simulink model "DBX_aero_parametric"  (R2015b)
settings: Solver=VariableStepAuto  StartTime=0.0  StopTime=10.0  RelTol=1e-3
undefined symbols (not defined in the file or in its folder): DBX_aero_param
libraries: simulink x28
settings Model: Creator=DTorres  LastModifiedBy=DTorres

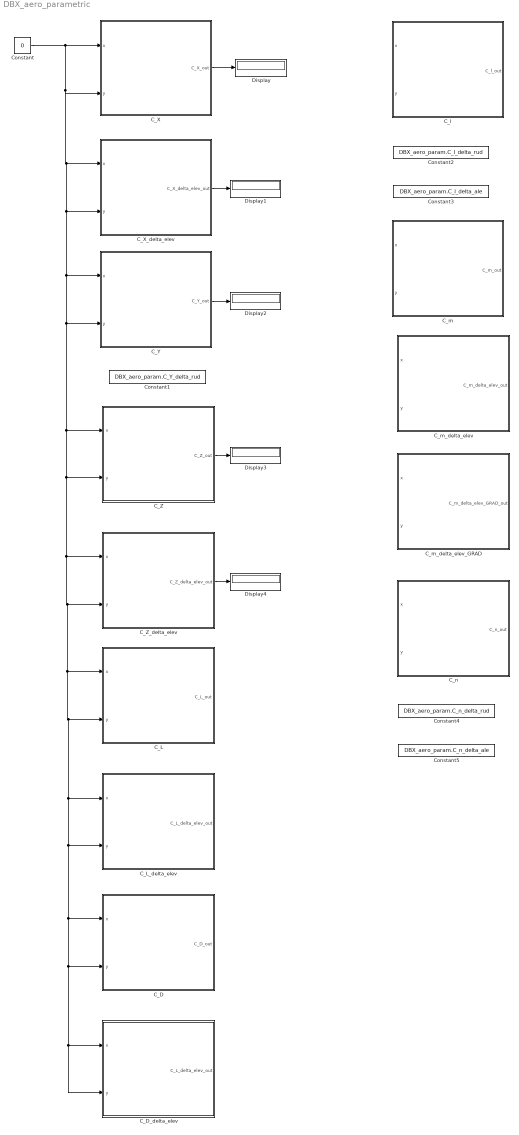
== system DBX_aero_parametric ==
  C_D : Subsystem
  C_D_delta_elev : Subsystem
  C_L : Subsystem
  C_L_delta_elev : Subsystem
  C_X : Subsystem
  C_X_delta_elev : Subsystem
  C_Y : Subsystem
  C_Z : Subsystem
  C_Z_delta_elev : Subsystem
  C_l : Subsystem
  C_m : Subsystem
  C_m_delta_elev : Subsystem
  C_m_delta_elev_GRAD : Subsystem
  C_n : Subsystem
  Constant : Constant  Value=0
  Constant1 : Constant  Value=DBX_aero_param.C_Y_delta_rud
  Constant2 : Constant  Value=DBX_aero_param.C_l_delta_rud
  Constant3 : Constant  Value=DBX_aero_param.C_l_delta_ale
  Constant4 : Constant  Value=DBX_aero_param.C_n_delta_rud
  Constant5 : Constant  Value=DBX_aero_param.C_n_delta_ale
  Display{,1..4} (5 alike) : Display
  wires:
  Constant/1 -> C_D_delta_elev/2(y), C_D_delta_elev/1(x), C_D/2(y), C_D/1(x), C_L_delta_elev/2(y), C_L_delta_elev/1(x), C_L/2(y), C_L/1(x), C_Z_delta_elev/2(y), C_Z_delta_elev/1(x), C_Z/2(y), C_Z/1(x), C_Y/2(y), C_Y/1(x), C_X_delta_elev/2(y), C_X_delta_elev/1(x), C_X/2(y), C_X/1(x)
  C_X/1(C_X_out) -> Display/1
  C_X_delta_elev/1(C_X_delta_elev_out) -> Display1/1
  C_Y/1(C_Y_out) -> Display2/1
  C_Z/1(C_Z_out) -> Display3/1
  C_Z_delta_elev/1(C_Z_delta_elev_out) -> Display4/1

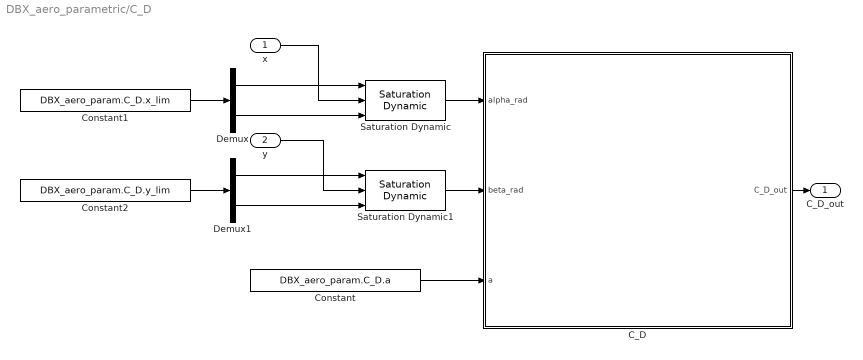
== system DBX_aero_parametric/C_D ==
  x : Inport
  y : Inport  Port=2
  C_D : MATLAB Function
  Constant : Constant  Value=DBX_aero_param.C_D.a
  Constant1 : Constant  Value=DBX_aero_param.C_D.x_lim
  Constant2 : Constant  Value=DBX_aero_param.C_D.y_lim
  Demux : Demux  Outputs=2
  Demux1 : Demux  Outputs=2
  Saturation Dynamic : simulink/Discontinuities/Saturation Dynamic  OutMin=[]  OutMax=[]  OutDataTypeStr=Inherit: Same as second input  OutDataType=fixdt(1, 16)  OutScaling=2^-10  DoSatur=off
  Saturation Dynamic1 : simulink/Discontinuities/Saturation Dynamic  OutMin=[]  OutMax=[]  OutDataTypeStr=Inherit: Same as second input  OutDataType=fixdt(1, 16)  OutScaling=2^-10  DoSatur=off
  C_D_out : Outport
  wires:
  Demux/1 -> Saturation Dynamic/1
  y/1 -> Saturation Dynamic1/2
  Demux/2 -> Saturation Dynamic/3
  Constant1/1 -> Demux/1
  x/1 -> Saturation Dynamic/2
  Demux1/2 -> Saturation Dynamic1/3
  Saturation Dynamic/1 -> C_D/1(alpha_rad)
  Demux1/1 -> Saturation Dynamic1/1
  Saturation Dynamic1/1 -> C_D/2(beta_rad)
  Constant2/1 -> Demux1/1
  C_D/1(C_D_out) -> C_D_out/1
  Constant/1 -> C_D/3(a)

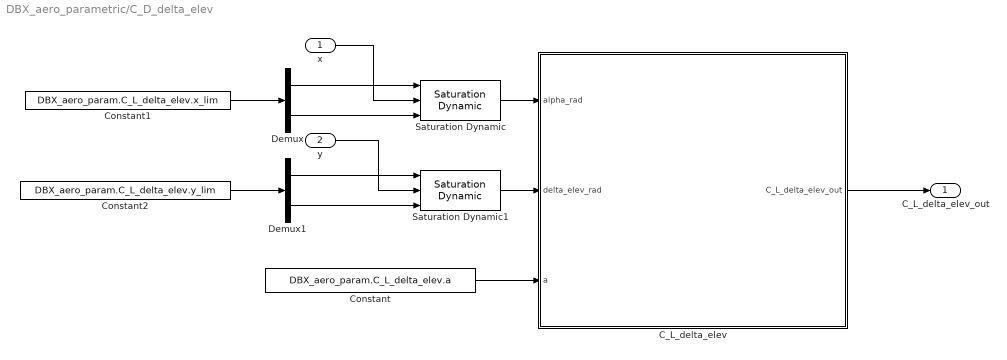
== system DBX_aero_parametric/C_D_delta_elev ==
  x : Inport
  y : Inport  Port=2
  C_L_delta_elev : MATLAB Function
  Constant : Constant  Value=DBX_aero_param.C_L_delta_elev.a
  Constant1 : Constant  Value=DBX_aero_param.C_L_delta_elev.x_lim
  Constant2 : Constant  Value=DBX_aero_param.C_L_delta_elev.y_lim
  Demux : Demux  Outputs=2
  Demux1 : Demux  Outputs=2
  Saturation Dynamic : simulink/Discontinuities/Saturation Dynamic  OutMin=[]  OutMax=[]  OutDataTypeStr=Inherit: Same as second input  OutDataType=fixdt(1, 16)  OutScaling=2^-10  DoSatur=off
  Saturation Dynamic1 : simulink/Discontinuities/Saturation Dynamic  OutMin=[]  OutMax=[]  OutDataTypeStr=Inherit: Same as second input  OutDataType=fixdt(1, 16)  OutScaling=2^-10  DoSatur=off
  C_L_delta_elev_out : Outport
  wires:
  Constant/1 -> C_L_delta_elev/3(a)
  C_L_delta_elev/1(C_L_delta_elev_out) -> C_L_delta_elev_out/1
  Constant2/1 -> Demux1/1
  Saturation Dynamic1/1 -> C_L_delta_elev/2(delta_elev_rad)
  Demux1/1 -> Saturation Dynamic1/1
  Saturation Dynamic/1 -> C_L_delta_elev/1(alpha_rad)
  Demux1/2 -> Saturation Dynamic1/3
  x/1 -> Saturation Dynamic/2
  Constant1/1 -> Demux/1
  Demux/2 -> Saturation Dynamic/3
  y/1 -> Saturation Dynamic1/2
  Demux/1 -> Saturation Dynamic/1

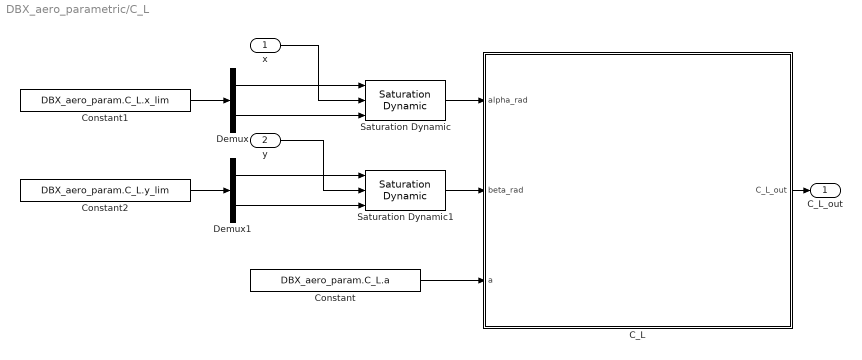
== system DBX_aero_parametric/C_L ==
  x : Inport
  y : Inport  Port=2
  C_L : MATLAB Function
  Constant : Constant  Value=DBX_aero_param.C_L.a
  Constant1 : Constant  Value=DBX_aero_param.C_L.x_lim
  Constant2 : Constant  Value=DBX_aero_param.C_L.y_lim
  Demux : Demux  Outputs=2
  Demux1 : Demux  Outputs=2
  Saturation Dynamic : simulink/Discontinuities/Saturation Dynamic  OutMin=[]  OutMax=[]  OutDataTypeStr=Inherit: Same as second input  OutDataType=fixdt(1, 16)  OutScaling=2^-10  DoSatur=off
  Saturation Dynamic1 : simulink/Discontinuities/Saturation Dynamic  OutMin=[]  OutMax=[]  OutDataTypeStr=Inherit: Same as second input  OutDataType=fixdt(1, 16)  OutScaling=2^-10  DoSatur=off
  C_L_out : Outport
  wires:
  Constant/1 -> C_L/3(a)
  C_L/1(C_L_out) -> C_L_out/1
  Constant2/1 -> Demux1/1
  Saturation Dynamic1/1 -> C_L/2(beta_rad)
  Demux1/1 -> Saturation Dynamic1/1
  Saturation Dynamic/1 -> C_L/1(alpha_rad)
  Demux1/2 -> Saturation Dynamic1/3
  x/1 -> Saturation Dynamic/2
  Constant1/1 -> Demux/1
  Demux/2 -> Saturation Dynamic/3
  y/1 -> Saturation Dynamic1/2
  Demux/1 -> Saturation Dynamic/1

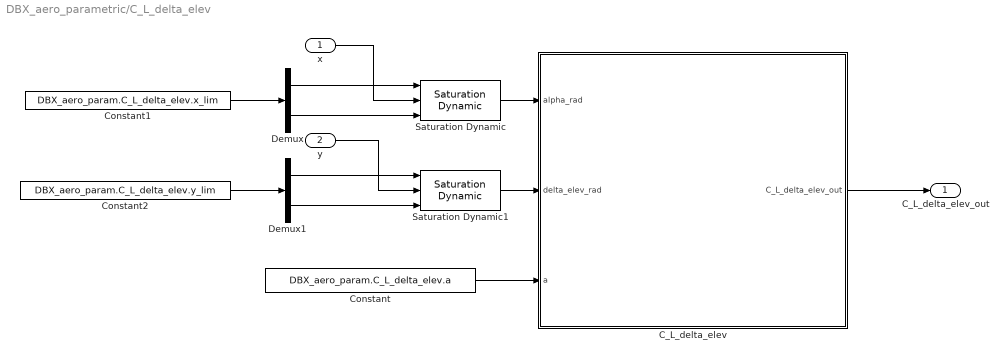
== system DBX_aero_parametric/C_L_delta_elev ==
  x : Inport
  y : Inport  Port=2
  C_L_delta_elev : MATLAB Function
  Constant : Constant  Value=DBX_aero_param.C_L_delta_elev.a
  Constant1 : Constant  Value=DBX_aero_param.C_L_delta_elev.x_lim
  Constant2 : Constant  Value=DBX_aero_param.C_L_delta_elev.y_lim
  Demux : Demux  Outputs=2
  Demux1 : Demux  Outputs=2
  Saturation Dynamic : simulink/Discontinuities/Saturation Dynamic  OutMin=[]  OutMax=[]  OutDataTypeStr=Inherit: Same as second input  OutDataType=fixdt(1, 16)  OutScaling=2^-10  DoSatur=off
  Saturation Dynamic1 : simulink/Discontinuities/Saturation Dynamic  OutMin=[]  OutMax=[]  OutDataTypeStr=Inherit: Same as second input  OutDataType=fixdt(1, 16)  OutScaling=2^-10  DoSatur=off
  C_L_delta_elev_out : Outport
  wires:
  Demux/1 -> Saturation Dynamic/1
  y/1 -> Saturation Dynamic1/2
  Demux/2 -> Saturation Dynamic/3
  Constant1/1 -> Demux/1
  x/1 -> Saturation Dynamic/2
  Demux1/2 -> Saturation Dynamic1/3
  Saturation Dynamic/1 -> C_L_delta_elev/1(alpha_rad)
  Demux1/1 -> Saturation Dynamic1/1
  Saturation Dynamic1/1 -> C_L_delta_elev/2(delta_elev_rad)
  Constant2/1 -> Demux1/1
  C_L_delta_elev/1(C_L_delta_elev_out) -> C_L_delta_elev_out/1
  Constant/1 -> C_L_delta_elev/3(a)

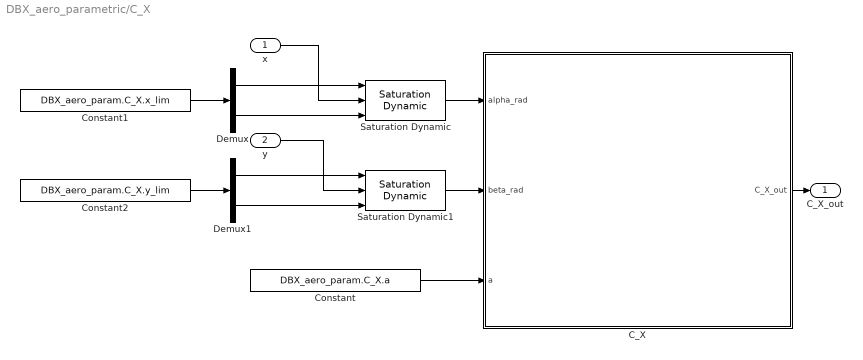
== system DBX_aero_parametric/C_X ==
  x : Inport
  y : Inport  Port=2
  C_X : MATLAB Function
  Constant : Constant  Value=DBX_aero_param.C_X.a
  Constant1 : Constant  Value=DBX_aero_param.C_X.x_lim
  Constant2 : Constant  Value=DBX_aero_param.C_X.y_lim
  Demux : Demux  Outputs=2
  Demux1 : Demux  Outputs=2
  Saturation Dynamic : simulink/Discontinuities/Saturation Dynamic  OutMin=[]  OutMax=[]  OutDataTypeStr=Inherit: Same as second input  OutDataType=fixdt(1, 16)  OutScaling=2^-10  DoSatur=off
  Saturation Dynamic1 : simulink/Discontinuities/Saturation Dynamic  OutMin=[]  OutMax=[]  OutDataTypeStr=Inherit: Same as second input  OutDataType=fixdt(1, 16)  OutScaling=2^-10  DoSatur=off
  C_X_out : Outport
  wires:
  Constant/1 -> C_X/3(a)
  C_X/1(C_X_out) -> C_X_out/1
  Constant2/1 -> Demux1/1
  Saturation Dynamic1/1 -> C_X/2(beta_rad)
  Demux1/1 -> Saturation Dynamic1/1
  Saturation Dynamic/1 -> C_X/1(alpha_rad)
  Demux1/2 -> Saturation Dynamic1/3
  x/1 -> Saturation Dynamic/2
  Constant1/1 -> Demux/1
  Demux/2 -> Saturation Dynamic/3
  y/1 -> Saturation Dynamic1/2
  Demux/1 -> Saturation Dynamic/1

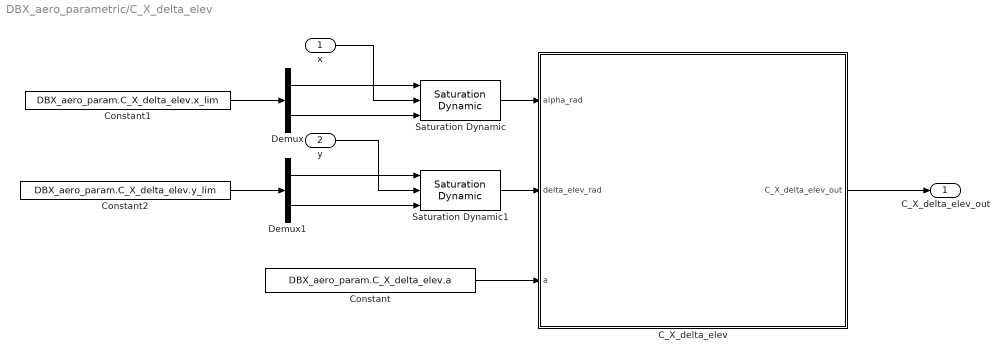
== system DBX_aero_parametric/C_X_delta_elev ==
  x : Inport
  y : Inport  Port=2
  C_X_delta_elev : MATLAB Function
  Constant : Constant  Value=DBX_aero_param.C_X_delta_elev.a
  Constant1 : Constant  Value=DBX_aero_param.C_X_delta_elev.x_lim
  Constant2 : Constant  Value=DBX_aero_param.C_X_delta_elev.y_lim
  Demux : Demux  Outputs=2
  Demux1 : Demux  Outputs=2
  Saturation Dynamic : simulink/Discontinuities/Saturation Dynamic  OutMin=[]  OutMax=[]  OutDataTypeStr=Inherit: Same as second input  OutDataType=fixdt(1, 16)  OutScaling=2^-10  DoSatur=off
  Saturation Dynamic1 : simulink/Discontinuities/Saturation Dynamic  OutMin=[]  OutMax=[]  OutDataTypeStr=Inherit: Same as second input  OutDataType=fixdt(1, 16)  OutScaling=2^-10  DoSatur=off
  C_X_delta_elev_out : Outport
  wires:
  Demux/1 -> Saturation Dynamic/1
  y/1 -> Saturation Dynamic1/2
  Demux/2 -> Saturation Dynamic/3
  Constant1/1 -> Demux/1
  x/1 -> Saturation Dynamic/2
  Demux1/2 -> Saturation Dynamic1/3
  Saturation Dynamic/1 -> C_X_delta_elev/1(alpha_rad)
  Demux1/1 -> Saturation Dynamic1/1
  Saturation Dynamic1/1 -> C_X_delta_elev/2(delta_elev_rad)
  Constant2/1 -> Demux1/1
  C_X_delta_elev/1(C_X_delta_elev_out) -> C_X_delta_elev_out/1
  Constant/1 -> C_X_delta_elev/3(a)

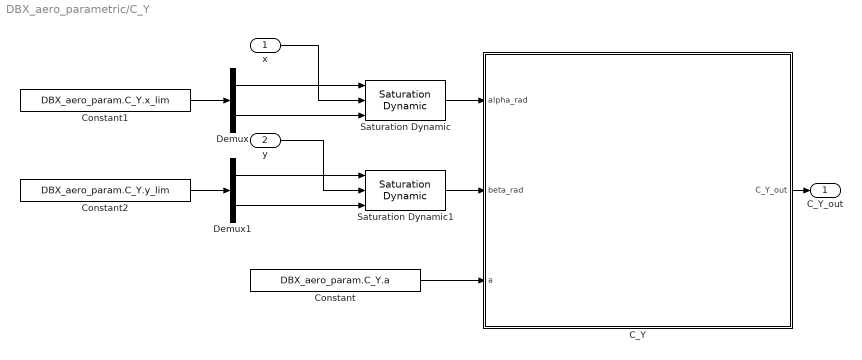
== system DBX_aero_parametric/C_Y ==
  x : Inport
  y : Inport  Port=2
  C_Y : MATLAB Function
  Constant : Constant  Value=DBX_aero_param.C_Y.a
  Constant1 : Constant  Value=DBX_aero_param.C_Y.x_lim
  Constant2 : Constant  Value=DBX_aero_param.C_Y.y_lim
  Demux : Demux  Outputs=2
  Demux1 : Demux  Outputs=2
  Saturation Dynamic : simulink/Discontinuities/Saturation Dynamic  OutMin=[]  OutMax=[]  OutDataTypeStr=Inherit: Same as second input  OutDataType=fixdt(1, 16)  OutScaling=2^-10  DoSatur=off
  Saturation Dynamic1 : simulink/Discontinuities/Saturation Dynamic  OutMin=[]  OutMax=[]  OutDataTypeStr=Inherit: Same as second input  OutDataType=fixdt(1, 16)  OutScaling=2^-10  DoSatur=off
  C_Y_out : Outport
  wires:
  Demux/1 -> Saturation Dynamic/1
  y/1 -> Saturation Dynamic1/2
  Demux/2 -> Saturation Dynamic/3
  Constant1/1 -> Demux/1
  x/1 -> Saturation Dynamic/2
  Demux1/2 -> Saturation Dynamic1/3
  Saturation Dynamic/1 -> C_Y/1(alpha_rad)
  Demux1/1 -> Saturation Dynamic1/1
  Saturation Dynamic1/1 -> C_Y/2(beta_rad)
  Constant2/1 -> Demux1/1
  C_Y/1(C_Y_out) -> C_Y_out/1
  Constant/1 -> C_Y/3(a)

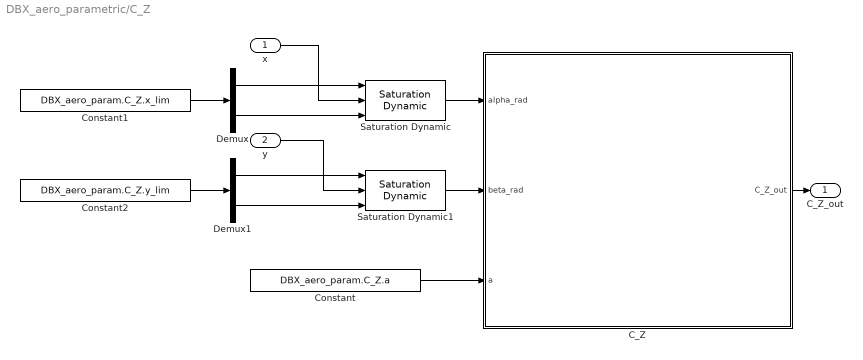
== system DBX_aero_parametric/C_Z ==
  x : Inport
  y : Inport  Port=2
  C_Z : MATLAB Function
  Constant : Constant  Value=DBX_aero_param.C_Z.a
  Constant1 : Constant  Value=DBX_aero_param.C_Z.x_lim
  Constant2 : Constant  Value=DBX_aero_param.C_Z.y_lim
  Demux : Demux  Outputs=2
  Demux1 : Demux  Outputs=2
  Saturation Dynamic : simulink/Discontinuities/Saturation Dynamic  OutMin=[]  OutMax=[]  OutDataTypeStr=Inherit: Same as second input  OutDataType=fixdt(1, 16)  OutScaling=2^-10  DoSatur=off
  Saturation Dynamic1 : simulink/Discontinuities/Saturation Dynamic  OutMin=[]  OutMax=[]  OutDataTypeStr=Inherit: Same as second input  OutDataType=fixdt(1, 16)  OutScaling=2^-10  DoSatur=off
  C_Z_out : Outport
  wires:
  Demux/1 -> Saturation Dynamic/1
  y/1 -> Saturation Dynamic1/2
  Demux/2 -> Saturation Dynamic/3
  Constant1/1 -> Demux/1
  x/1 -> Saturation Dynamic/2
  Demux1/2 -> Saturation Dynamic1/3
  Saturation Dynamic/1 -> C_Z/1(alpha_rad)
  Demux1/1 -> Saturation Dynamic1/1
  Saturation Dynamic1/1 -> C_Z/2(beta_rad)
  Constant2/1 -> Demux1/1
  C_Z/1(C_Z_out) -> C_Z_out/1
  Constant/1 -> C_Z/3(a)

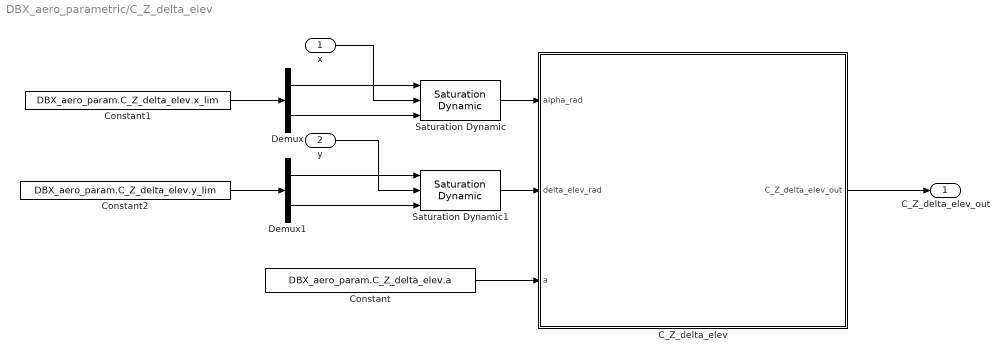
== system DBX_aero_parametric/C_Z_delta_elev ==
  x : Inport
  y : Inport  Port=2
  C_Z_delta_elev : MATLAB Function
  Constant : Constant  Value=DBX_aero_param.C_Z_delta_elev.a
  Constant1 : Constant  Value=DBX_aero_param.C_Z_delta_elev.x_lim
  Constant2 : Constant  Value=DBX_aero_param.C_Z_delta_elev.y_lim
  Demux : Demux  Outputs=2
  Demux1 : Demux  Outputs=2
  Saturation Dynamic : simulink/Discontinuities/Saturation Dynamic  OutMin=[]  OutMax=[]  OutDataTypeStr=Inherit: Same as second input  OutDataType=fixdt(1, 16)  OutScaling=2^-10  DoSatur=off
  Saturation Dynamic1 : simulink/Discontinuities/Saturation Dynamic  OutMin=[]  OutMax=[]  OutDataTypeStr=Inherit: Same as second input  OutDataType=fixdt(1, 16)  OutScaling=2^-10  DoSatur=off
  C_Z_delta_elev_out : Outport
  wires:
  Constant/1 -> C_Z_delta_elev/3(a)
  C_Z_delta_elev/1(C_Z_delta_elev_out) -> C_Z_delta_elev_out/1
  Constant2/1 -> Demux1/1
  Saturation Dynamic1/1 -> C_Z_delta_elev/2(delta_elev_rad)
  Demux1/1 -> Saturation Dynamic1/1
  Saturation Dynamic/1 -> C_Z_delta_elev/1(alpha_rad)
  Demux1/2 -> Saturation Dynamic1/3
  x/1 -> Saturation Dynamic/2
  Constant1/1 -> Demux/1
  Demux/2 -> Saturation Dynamic/3
  y/1 -> Saturation Dynamic1/2
  Demux/1 -> Saturation Dynamic/1

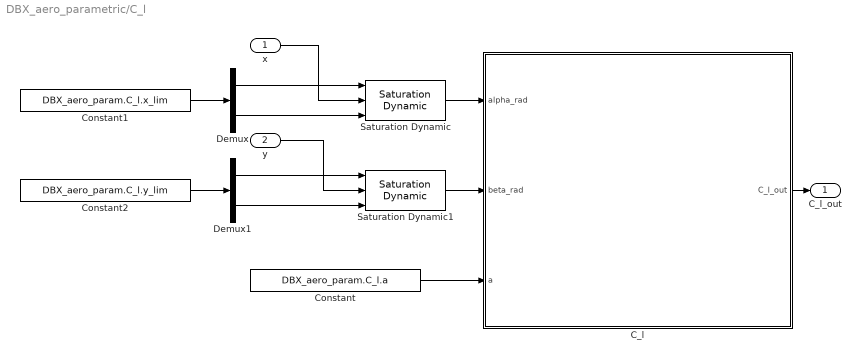
== system DBX_aero_parametric/C_l ==
  x : Inport
  y : Inport  Port=2
  C_l : MATLAB Function
  Constant : Constant  Value=DBX_aero_param.C_l.a
  Constant1 : Constant  Value=DBX_aero_param.C_l.x_lim
  Constant2 : Constant  Value=DBX_aero_param.C_l.y_lim
  Demux : Demux  Outputs=2
  Demux1 : Demux  Outputs=2
  Saturation Dynamic : simulink/Discontinuities/Saturation Dynamic  OutMin=[]  OutMax=[]  OutDataTypeStr=Inherit: Same as second input  OutDataType=fixdt(1, 16)  OutScaling=2^-10  DoSatur=off
  Saturation Dynamic1 : simulink/Discontinuities/Saturation Dynamic  OutMin=[]  OutMax=[]  OutDataTypeStr=Inherit: Same as second input  OutDataType=fixdt(1, 16)  OutScaling=2^-10  DoSatur=off
  C_l_out : Outport
  wires:
  Demux/1 -> Saturation Dynamic/1
  y/1 -> Saturation Dynamic1/2
  Demux/2 -> Saturation Dynamic/3
  Constant1/1 -> Demux/1
  x/1 -> Saturation Dynamic/2
  Demux1/2 -> Saturation Dynamic1/3
  Saturation Dynamic/1 -> C_l/1(alpha_rad)
  Demux1/1 -> Saturation Dynamic1/1
  Saturation Dynamic1/1 -> C_l/2(beta_rad)
  Constant2/1 -> Demux1/1
  C_l/1(C_l_out) -> C_l_out/1
  Constant/1 -> C_l/3(a)

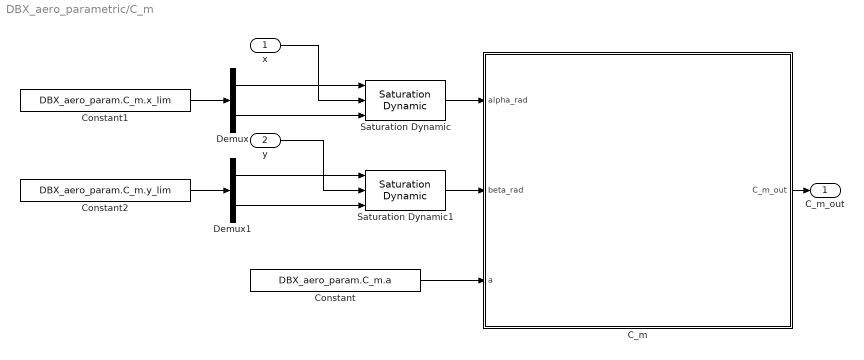
== system DBX_aero_parametric/C_m ==
  x : Inport
  y : Inport  Port=2
  C_m : MATLAB Function
  Constant : Constant  Value=DBX_aero_param.C_m.a
  Constant1 : Constant  Value=DBX_aero_param.C_m.x_lim
  Constant2 : Constant  Value=DBX_aero_param.C_m.y_lim
  Demux : Demux  Outputs=2
  Demux1 : Demux  Outputs=2
  Saturation Dynamic : simulink/Discontinuities/Saturation Dynamic  OutMin=[]  OutMax=[]  OutDataTypeStr=Inherit: Same as second input  OutDataType=fixdt(1, 16)  OutScaling=2^-10  DoSatur=off
  Saturation Dynamic1 : simulink/Discontinuities/Saturation Dynamic  OutMin=[]  OutMax=[]  OutDataTypeStr=Inherit: Same as second input  OutDataType=fixdt(1, 16)  OutScaling=2^-10  DoSatur=off
  C_m_out : Outport
  wires:
  Demux/1 -> Saturation Dynamic/1
  y/1 -> Saturation Dynamic1/2
  Demux/2 -> Saturation Dynamic/3
  Constant1/1 -> Demux/1
  x/1 -> Saturation Dynamic/2
  Demux1/2 -> Saturation Dynamic1/3
  Saturation Dynamic/1 -> C_m/1(alpha_rad)
  Demux1/1 -> Saturation Dynamic1/1
  Saturation Dynamic1/1 -> C_m/2(beta_rad)
  Constant2/1 -> Demux1/1
  C_m/1(C_m_out) -> C_m_out/1
  Constant/1 -> C_m/3(a)

== system DBX_aero_parametric/C_m_delta_elev ==
  x : Inport
  y : Inport  Port=2
  C_m_delta_elev : MATLAB Function
  Constant : Constant  Value=DBX_aero_param.C_m_delta_elev.a
  Constant1 : Constant  Value=DBX_aero_param.C_m_delta_elev.x_lim
  Constant2 : Constant  Value=DBX_aero_param.C_m_delta_elev.y_lim
  Demux : Demux  Outputs=2
  Demux1 : Demux  Outputs=2
  Saturation Dynamic : simulink/Discontinuities/Saturation Dynamic  OutMin=[]  OutMax=[]  OutDataTypeStr=Inherit: Same as second input  OutDataType=fixdt(1, 16)  OutScaling=2^-10  DoSatur=off
  Saturation Dynamic1 : simulink/Discontinuities/Saturation Dynamic  OutMin=[]  OutMax=[]  OutDataTypeStr=Inherit: Same as second input  OutDataType=fixdt(1, 16)  OutScaling=2^-10  DoSatur=off
  C_m_delta_elev_out : Outport
  wires:
  Constant/1 -> C_m_delta_elev/3(a)
  C_m_delta_elev/1(C_m_delta_elev_out) -> C_m_delta_elev_out/1
  Constant2/1 -> Demux1/1
  Saturation Dynamic1/1 -> C_m_delta_elev/2(delta_elev_rad)
  Demux1/1 -> Saturation Dynamic1/1
  Saturation Dynamic/1 -> C_m_delta_elev/1(alpha_rad)
  Demux1/2 -> Saturation Dynamic1/3
  x/1 -> Saturation Dynamic/2
  Constant1/1 -> Demux/1
  Demux/2 -> Saturation Dynamic/3
  y/1 -> Saturation Dynamic1/2
  Demux/1 -> Saturation Dynamic/1

== system DBX_aero_parametric/C_m_delta_elev_GRAD ==
  x : Inport
  y : Inport  Port=2
  C_m_delta_elev_GRAD : MATLAB Function
  Constant : Constant  Value=DBX_aero_param.C_m_delta_elev_GRAD.a
  Constant1 : Constant  Value=DBX_aero_param.C_m_delta_elev_GRAD.x_lim
  Constant2 : Constant  Value=DBX_aero_param.C_m_delta_elev_GRAD.y_lim
  Demux : Demux  Outputs=2
  Demux1 : Demux  Outputs=2
  Saturation Dynamic : simulink/Discontinuities/Saturation Dynamic  OutMin=[]  OutMax=[]  OutDataTypeStr=Inherit: Same as second input  OutDataType=fixdt(1, 16)  OutScaling=2^-10  DoSatur=off
  Saturation Dynamic1 : simulink/Discontinuities/Saturation Dynamic  OutMin=[]  OutMax=[]  OutDataTypeStr=Inherit: Same as second input  OutDataType=fixdt(1, 16)  OutScaling=2^-10  DoSatur=off
  C_m_delta_elev_GRAD_out : Outport
  wires:
  Demux/1 -> Saturation Dynamic/1
  y/1 -> Saturation Dynamic1/2
  Demux/2 -> Saturation Dynamic/3
  Constant1/1 -> Demux/1
  x/1 -> Saturation Dynamic/2
  Demux1/2 -> Saturation Dynamic1/3
  Saturation Dynamic/1 -> C_m_delta_elev_GRAD/1(alpha_rad)
  Demux1/1 -> Saturation Dynamic1/1
  Saturation Dynamic1/1 -> C_m_delta_elev_GRAD/2(delta_elev_rad)
  Constant2/1 -> Demux1/1
  C_m_delta_elev_GRAD/1(C_m_delta_elev_GRAD_out) -> C_m_delta_elev_GRAD_out/1
  Constant/1 -> C_m_delta_elev_GRAD/3(a)

== system DBX_aero_parametric/C_n ==
  x : Inport
  y : Inport  Port=2
  C_n : MATLAB Function
  Constant : Constant  Value=DBX_aero_param.C_n.a
  Constant1 : Constant  Value=DBX_aero_param.C_n.x_lim
  Constant2 : Constant  Value=DBX_aero_param.C_n.y_lim
  Demux : Demux  Outputs=2
  Demux1 : Demux  Outputs=2
  Saturation Dynamic : simulink/Discontinuities/Saturation Dynamic  OutMin=[]  OutMax=[]  OutDataTypeStr=Inherit: Same as second input  OutDataType=fixdt(1, 16)  OutScaling=2^-10  DoSatur=off
  Saturation Dynamic1 : simulink/Discontinuities/Saturation Dynamic  OutMin=[]  OutMax=[]  OutDataTypeStr=Inherit: Same as second input  OutDataType=fixdt(1, 16)  OutScaling=2^-10  DoSatur=off
  C_n_out : Outport
  wires:
  Demux/1 -> Saturation Dynamic/1
  y/1 -> Saturation Dynamic1/2
  Demux/2 -> Saturation Dynamic/3
  Constant1/1 -> Demux/1
  x/1 -> Saturation Dynamic/2
  Demux1/2 -> Saturation Dynamic1/3
  Saturation Dynamic/1 -> C_n/1(alpha_rad)
  Demux1/1 -> Saturation Dynamic1/1
  Saturation Dynamic1/1 -> C_n/2(beta_rad)
  Constant2/1 -> Demux1/1
  C_n/1(C_n_out) -> C_n_out/1
  Constant/1 -> C_n/3(a)

== matlab function DBX_aero_parametric/C_X_delta_elev/C_X_delta_elev ==
  data: alpha_rad input; delta_elev_rad input; a input; C_X_delta_elev_out output
function C_X_delta_elev_out   = DBX_aero_C_X_delta_elev(alpha_rad,delta_elev_rad,a)
% % C_X_delta_elev(alpha,delta_elev) = (a_0+a_1*alpha_rad+a_2*alpha_rad^2+a_3*alpha_rad^3+a_4*alpha_rad^4) + a_5*delta_elev_rad + a_6*delta_elev_rad^2



C_X_delta_elev_out     =    (a(1)+a(2)*alpha_rad+a(3)*alpha_rad^2+a(4)*alpha_rad^3+a(5)*alpha_rad^4) + a(6)*delta_elev_rad + a(7)*delta_elev_rad^2;

end

== matlab function DBX_aero_parametric/C_X/C_X ==
  data: alpha_rad input; beta_rad input; a input; C_X_out output
function C_X_out   = DBX_aero_C_X(alpha_rad,beta_rad,a)
%% C_X(alpha,beta) = (a(1)+a(2)*alpha_rad+a(3)*alpha_rad^2+a(4)*alpha_rad^3+a(5)*alpha_rad^4)*(1-beta_rad^2)



C_X_out     =    (a(1)+a(2)*alpha_rad+a(3)*alpha_rad^2+a(4)*alpha_rad^3+a(5)*alpha_rad^4)*(1-beta_rad^2);

end

== matlab function DBX_aero_parametric/C_Y/C_Y ==
  data: alpha_rad input; beta_rad input; a input; C_Y_out output
function C_Y_out   = DBX_aero_C_Y(alpha_rad,beta_rad,a)
%% C_Y(alpha,beta) = a_1*beta_rad + a_2*alpha_rad + a_3*beta_rad^2 + a_4*alpha_rad^2 + a_5*alpha_rad*beta_rad


C_Y_out     =    a(1)*beta_rad + a(2)*alpha_rad + a(3)*beta_rad^2 + a(4)*alpha_rad^2 + a(5)*alpha_rad*beta_rad;

end

== matlab function DBX_aero_parametric/C_Z/C_Z ==
  data: alpha_rad input; beta_rad input; a input; C_Z_out output
function C_Z_out   = DBX_aero_C_Z(alpha_rad,beta_rad,a)
%% C_Z(alpha,beta) = (a(1)+a(2)*alpha_rad+a(3)*alpha_rad^2+a(4)*alpha_rad^3+a(5)*alpha_rad^4)*(1-beta_rad^2)



C_Z_out     =    (a(1)+a(2)*alpha_rad+a(3)*alpha_rad^2+a(4)*alpha_rad^3+a(5)*alpha_rad^4)*(1-beta_rad^2);

end

== matlab function DBX_aero_parametric/C_Z_delta_elev/C_Z_delta_elev ==
  data: alpha_rad input; delta_elev_rad input; a input; C_Z_delta_elev_out output
function C_Z_delta_elev_out   = DBX_aero_C_Z_delta_elev(alpha_rad,delta_elev_rad,a)
% % C_Z_delta_elev(alpha,delta_elev) = (a_0+a_1*alpha_rad+a_2*alpha_rad^2+a_3*alpha_rad^3+a_4*alpha_rad^4) + a_5*delta_elev_rad + a_6*delta_elev_rad^2



C_Z_delta_elev_out     =    (a(1)+a(2)*alpha_rad+a(3)*alpha_rad^2+a(4)*alpha_rad^3+a(5)*alpha_rad^4) + a(6)*delta_elev_rad + a(7)*delta_elev_rad^2;

end

== matlab function DBX_aero_parametric/C_L/C_L ==
  data: alpha_rad input; beta_rad input; a input; C_L_out output
function C_L_out   = DBX_aero_C_L(alpha_rad,beta_rad,a)
%% C_D(alpha,beta) = (a(1)+a(2)*alpha_rad+a(3)*alpha_rad^2+a(4)*alpha_rad^3+a(5)*alpha_rad^4)*(1-beta_rad^2)



C_L_out     =    (a(1)+a(2)*alpha_rad+a(3)*alpha_rad^2+a(4)*alpha_rad^3+a(5)*alpha_rad^4)*(1-beta_rad^2);

end

== matlab function DBX_aero_parametric/C_L_delta_elev/C_L_delta_elev ==
  data: alpha_rad input; delta_elev_rad input; a input; C_L_delta_elev_out output
function C_L_delta_elev_out   = DBX_aero_C_L_delta_elev(alpha_rad,delta_elev_rad,a)
% % C_L_delta_elev(alpha,delta_elev) = (a_0+a_1*alpha_rad+a_2*alpha_rad^2+a_3*alpha_rad^3+a_4*alpha_rad^4) + a_5*delta_elev_rad + a_6*delta_elev_rad^2

C_L_delta_elev_out     =    (a(1)+a(2)*alpha_rad+a(3)*alpha_rad^2+a(4)*alpha_rad^3+a(5)*alpha_rad^4) + a(6)*delta_elev_rad + a(7)*delta_elev_rad^2;

end

== matlab function DBX_aero_parametric/C_D/C_D ==
  data: alpha_rad input; beta_rad input; a input; C_D_out output
function C_D_out   = DBX_aero_C_D(alpha_rad,beta_rad,a)
%% C_D(alpha,beta) = (a(1)+a(2)*alpha_rad+a(3)*alpha_rad^2+a(4)*alpha_rad^3+a(5)*alpha_rad^4)*(1-beta_rad^2)

C_D_out     =    (a(1)+a(2)*alpha_rad+a(3)*alpha_rad^2+a(4)*alpha_rad^3+a(5)*alpha_rad^4)*(1-beta_rad^2);

end

== matlab function DBX_aero_parametric/C_D_delta_elev/C_L_delta_elev ==
  data: alpha_rad input; delta_elev_rad input; a input; C_L_delta_elev_out output
function C_L_delta_elev_out   = DBX_aero_C_L_delta_elev(alpha_rad,delta_elev_rad,a)
% % C_L_delta_elev(alpha,delta_elev) = (a_0+a_1*alpha_rad+a_2*alpha_rad^2+a_3*alpha_rad^3+a_4*alpha_rad^4) + a_5*delta_elev_rad + a_6*delta_elev_rad^2

C_L_delta_elev_out     =    (a(1)+a(2)*alpha_rad+a(3)*alpha_rad^2+a(4)*alpha_rad^3+a(5)*alpha_rad^4) + a(6)*delta_elev_rad + a(7)*delta_elev_rad^2;

end

== matlab function DBX_aero_parametric/C_l/C_l ==
  data: alpha_rad input; beta_rad input; a input; C_l_out output
function C_l_out   = DBX_aero_C_l(alpha_rad,beta_rad,a)
%% C_l(alpha,beta) =  a_1*beta_rad+a_2*beta_rad*alpha_rad+a_3*alpha_rad^2*beta_rad+a_4*beta_rad^2+a_5*alpha_rad*beta_rad^2+a_6*alpha_rad^3*beta_rad+a_7*alpha_rad^4*beta_rad+a_8*alpha_rad^2*beta_rad^2


C_l_out     =     a(1)*beta_rad+a(2)*beta_rad*alpha_rad+a(3)*alpha_rad^2*beta_rad+a(4)*beta_rad^2+a(5)*alpha_rad*beta_rad^2+a(6)*alpha_rad^3*beta_rad+a(7)*alpha_rad^4*beta_rad+a(8)*alpha_rad^2*beta_rad^2;

end

== matlab function DBX_aero_parametric/C_m/C_m ==
  data: alpha_rad input; beta_rad input; a input; C_m_out output
function C_m_out   = DBX_aero_C_m(alpha_rad,beta_rad,a)
%% C_m(alpha,beta) = (a(1)+a(2)*alpha_rad+a(3)*alpha_rad^2+a(4)*alpha_rad^3+a(5)*alpha_rad^4)*(1-beta_rad^2)

C_m_out     =    (a(1)+a(2)*alpha_rad+a(3)*alpha_rad^2+a(4)*alpha_rad^3+a(5)*alpha_rad^4)*(1-beta_rad^2);

end

== matlab function DBX_aero_parametric/C_m_delta_elev/C_m_delta_elev ==
  data: alpha_rad input; delta_elev_rad input; a input; C_m_delta_elev_out output
function C_m_delta_elev_out   = DBX_aero_C_m_delta_elev(alpha_rad,delta_elev_rad,a)
% %  C_m_delta_elev(alpha,delta_elev) = a_1*alpha_rad+a_2*delta_elev_rad+a_3*alpha_rad*delta_elev_rad+a_4*delta_elev_rad^2+a_5*alpha_rad^2*delta_elev_rad+a_6*delta_elev_rad^3+a_7*alpha_rad*delta_elev_rad^2

C_m_delta_elev_out     =     a(1)*alpha_rad+a(2)*delta_elev_rad+a(3)*alpha_rad*delta_elev_rad+a(4)*delta_elev_rad^2+a(5)*alpha_rad^2*delta_elev_rad+a(6)*delta_elev_rad^3+a(7)*alpha_rad*delta_elev_rad^2 ; 

end

== matlab function DBX_aero_parametric/C_m_delta_elev_GRAD/C_m_delta_elev_GRAD ==
  data: alpha_rad input; delta_elev_rad input; a input; C_m_delta_elev_GRAD_out output
function C_m_delta_elev_GRAD_out   = DBX_aero_C_m_delta_elev_GRAD(alpha_rad,delta_elev_rad,a)
% %  C_m_delta_elev_GRAD(alpha,delta_elev) = a_1*alpha_rad+a_2+a_3*alpha_rad+a_4*delta_elev_rad+a_5*alpha_rad^2*+a_6*delta_elev_rad^2+a_7*alpha_rad*delta_elev_rad

C_m_delta_elev_GRAD_out     =     a(1)*alpha_rad+a(2)+a(3)*alpha_rad+a(4)*delta_elev_rad+a(5)*alpha_rad^2*+a(6)*delta_elev_rad^2+a(7)*alpha_rad*delta_elev_rad ; 

end

== matlab function DBX_aero_parametric/C_n/C_n ==
  data: alpha_rad input; beta_rad input; a input; C_n_out output
function C_n_out   = DBX_aero_C_n(alpha_rad,beta_rad,a)
%% C_n(alpha,beta) =   a_1*beta_rad+a_2*beta_rad*alpha_rad+a_3*alpha_rad^2*beta_rad+a_4*beta_rad^2+a_5*alpha_rad*beta_rad^2+a_6*alpha_rad^3*beta_rad+a_7*alpha_rad^4*beta_rad+a_8*alpha_rad^2*beta_rad^2


C_n_out     =      a(1)*beta_rad+a(2)*beta_rad*alpha_rad+a(3)*alpha_rad^2*beta_rad+a(4)*beta_rad^2+a(5)*alpha_rad*beta_rad^2+a(6)*alpha_rad^3*beta_rad+a(7)*alpha_rad^4*beta_rad+a(8)*alpha_rad^2*beta_rad^2;

end
